simulink model "chap11_4sim"  (Simulink 6.3)
settings: Solver=ode45  StartTime=0  StopTime=5  RelTol=1e-3
values from neighbouring files (symbols this model uses):
  b = 1    [chap11_4int.m]    (also in chap11_6int.m = 0.5)
  bc = 30.0    (= 30)    [chap11_4int.m]    (also in chap11_5int.m = 3)
  bc1 = bc/Gain    (= 0.454545454545)    [chap11_4int.m]
  Ce = 1.2    [chap11_2.m]    (also in chap11_3plant.m; chap11_4int.m = 0.001; chap11_5int.m = 0.001)
  Fc = 0.28    [chap11_1plant.m]    (also in chap11_2plant.m = 15; chap11_3plant.m = 15; chap11_4int.m = 100; chap11_5int.m = 10)
  Fc1 = Fc/Gain    (= 1.51515151515)    [chap11_4int.m]
  J = 1.0    (= 1)    [chap11_1plant.m]    (also in chap11_2.m = 0.6; chap11_3plant.m = 0.6; chap11_4int.m = 2; chap11_6int.m = 2)
  kd = 6    [chap11_4int.m]    (also in chap11_5int.m; chap11_6int.m)
  kdd = 1.5    [chap11_4int.m]    (also in chap11_5int.m = 50)
  ki = 0.001    [chap11_4int.m]    (also in chap11_5int.m)
  kii = 0.1    [chap11_4int.m]    (also in chap11_5int.m = 1)
  km = 1.0    (= 1)    [chap11_4int.m]    (also in chap11_5int.m = 10)
  kpp = 150    [chap11_4int.m]    (also in chap11_5int.m = 100)
  ku = 11    [chap11_4int.m]    (also in chap11_5int.m)
  kv = 2.0    (= 2)    [chap11_2plant.m]    (also in chap11_3plant.m; chap11_4int.m; chap11_5int.m; chap11_6int.m)
  L = 0.001    [chap11_4int.m]    (also in chap11_5int.m)
  R = 7.77    [chap11_2.m]    (also in chap11_3plant.m; chap11_4int.m = 1; chap11_5int.m = 1)
undefined symbols (not defined in the file or in its folder): sgn
libraries: simulink_extras x1
settings Model: LastModifiedBy=Administrator  ExtModeTrigMode=oneshot  ExtModeArmWhenConnect=off  StrictBusMsg=None
settings DataIOCC: LimitDataPoints=off
settings OptimizationCC: BlockReduction=off  BooleanDataType=off
settings DebuggingCC: SolverPrmCheckMsg=none
settings HardwareCC: TargetUnknown=on

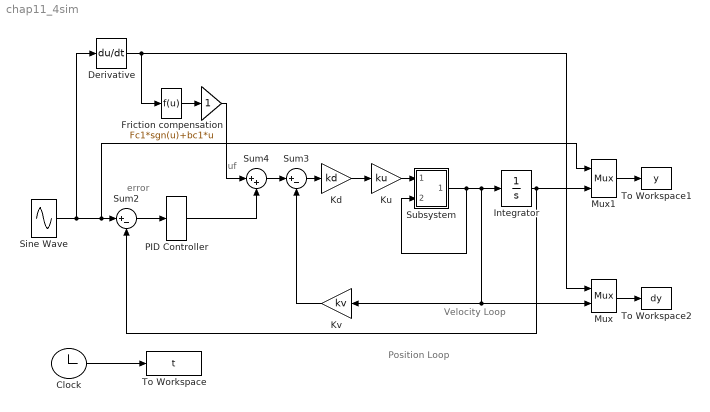
== system chap11_4sim ==
  note: uf
  note: Position Loop
  note: Velocity Loop
  note: error
  "     " : Gain  SaturateOnIntegerOverflow=on
  Clock : Clock
      settings: Decimation=10
  Derivative : Derivative
  Friction compensation : Fcn  Expr=Fc1*sgn(u)+bc1*u
  Integrator : Integrator
  Kd : Gain  Gain=kd  SaturateOnIntegerOverflow=on
  Ku : Gain  Gain=ku  SaturateOnIntegerOverflow=on
  Kv : Gain  Orientation=left  Gain=kv  SaturateOnIntegerOverflow=on
  Mux : Mux  Inputs=2
  Mux1 : Mux  Inputs=2
  PID Controller : simulink_extras/Additional Linear/PID Controller  P=kpp  I=kii  D=kdd
  Sine Wave : Sin  SampleTime=0
  Subsystem : Subsystem
  Sum2 : Sum  Inputs=|+-  SaturateOnIntegerOverflow=on  InputSameDT=on
  Sum3 : Sum  Inputs=|+-  SaturateOnIntegerOverflow=on  InputSameDT=on
  Sum4 : Sum  Inputs=|++  SaturateOnIntegerOverflow=on  InputSameDT=on
  To Workspace : ToWorkspace  VariableName=t  SampleTime=-1  SaveFormat=Array
  To Workspace1 : ToWorkspace  VariableName=y  SampleTime=-1  SaveFormat=Array
  To Workspace2 : ToWorkspace  VariableName=dy  SampleTime=-1  SaveFormat=Array
  wires:
  Sum3/1 -> Kd/1
  Mux/1 -> To Workspace2/1
  Mux1/1 -> To Workspace1/1
  Subsystem/1(Out1) -> Integrator/1, Kv/1, Mux/2, Subsystem/2(In2)
  Integrator/1 -> Mux1/2, Sum2/2
  Sum2/1 -> PID Controller/1
  Friction compensation/1 -> "     "/1
  "     "/1 -> Sum4/1
  Kv/1 -> Sum3/2
  PID Controller/1 -> Sum4/2
  Sum4/1 -> Sum3/1
  Ku/1 -> Subsystem/1(In1)
  Kd/1 -> Ku/1
  Sine Wave/1 -> Mux1/1, Sum2/1, Derivative/1
  Clock/1 -> To Workspace/1
  Derivative/1 -> Mux/1, Friction compensation/1

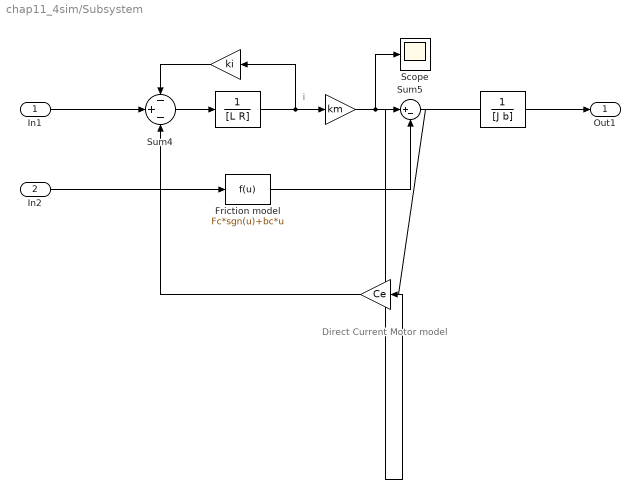
== system chap11_4sim/Subsystem ==
  note: i
  note: Direct Current Motor model
  In1 : Inport
  In2 : Inport  Port=2
  "    " : Gain  Orientation=left  Gain=Ce  SaturateOnIntegerOverflow=on
  "      " : Gain  Orientation=left  Gain=ki  SaturateOnIntegerOverflow=on
  "  " : Gain  Gain=km  SaturateOnIntegerOverflow=on
  "   " : TransferFcn  Denominator=[L R]
  "    " : TransferFcn  Denominator=[J b]
  Friction model : Fcn  Expr=Fc*sgn(u)+bc*u
  Scope : Scope
      settings: YMin=-80  YMax=80  MaxDataPoints=50000
  Sum4 : Sum  Inputs=-+-  InputSameDT=on
  Sum5 : Sum  Inputs=|+-  SaturateOnIntegerOverflow=on  InputSameDT=on
  Out1 : Outport
  wires:
  Sum5/1 -> "    "/1
  "    "/1 -> Sum4/3
  "    "/1 -> "    "/1, Out1/1
  "   "/1 -> "      "/1, "  "/1
  "      "/1 -> Sum4/1
  "  "/1 -> Sum5/1, Scope/1
  Friction model/1 -> Sum5/2
  In1/1 -> Sum4/2
  In2/1 -> Friction model/1
  Sum4/1 -> "   "/1
